simulink model "SAF"  (R2013a)
settings: Solver=ode3  StartTime=0.0  StopTime=0.5  RelTol=1e-3
InitFcn:
  | Ts=5e-6;
libraries: powerlib x25, dsparch4 x1
settings Model: Creator=smartworld  LastModifiedBy=Shubashini
settings DataIOCC: SignalLoggingSaveFormat=ModelDataLogs  InspectSignalLogs=on
settings OptimizationCC: ExpressionDepthLimit=2147483647
settings DebuggingCC: FcnCallInpInsideContextMsg=UseLocalSettings  StrictBusMsg=Warning
settings GRTTargetCC: CombineOutputUpdateFcns=off  GRTInterface=on

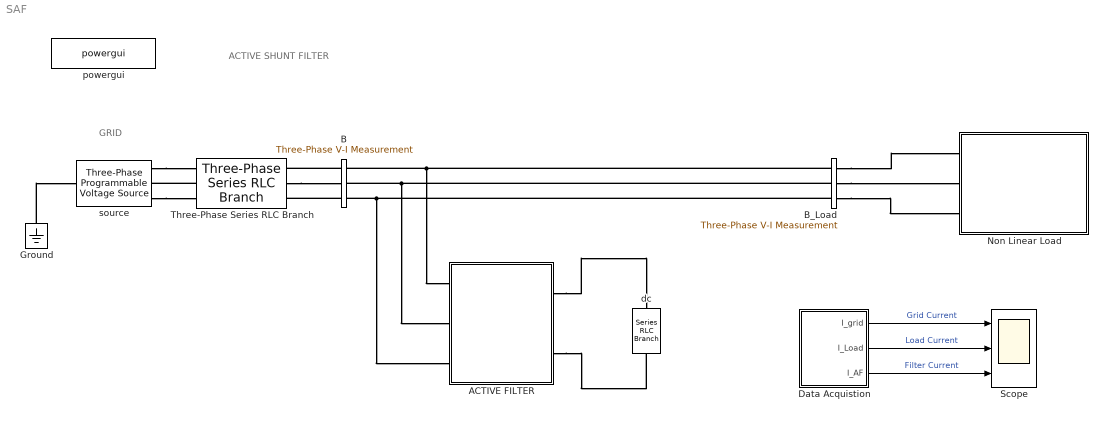
== system SAF ==
  note: ACTIVE SHUNT FILTER
  note: GRID
  ACTIVE FILTER : Subsystem
      mask Display: fprintf('ACTIVE\nFILTER')
  B : powerlib/Measurements/Three-Phase V-I Measurement  VoltageMeasurement=phase-to-ground  SetLabelV=on  LabelV=Vabc  Vpu=off  VpuLL=off  CurrentMeasurement=yes  SetLabelI=on  LabelI=Iabc  Ipu=off  Pbase=100e6  Vbase=500e3  OutputType=Complex  PhasorSimulation=off  PSBequivalent=0
  B_Load : powerlib/Measurements/Three-Phase V-I Measurement  VoltageMeasurement=phase-to-ground  SetLabelV=on  LabelV=Vabc_NL  Vpu=off  VpuLL=off  CurrentMeasurement=yes  SetLabelI=on  LabelI=Iabc_NL  Ipu=off  Pbase=100e6  Vbase=500e3  OutputType=Complex  PhasorSimulation=off  PSBequivalent=0
  Data Acquistion : Subsystem
  Ground : powerlib/Elements/Ground  LConnTagsString=a
  Non Linear Load : Subsystem
      mask Display: fprintf('Non Linear\nLoad')
  Scope : Scope  NumInputPorts=3
      settings: TimeRange=0.5  YMin=-4~-4~-2  YMax=4~4~2  SaveName=Current_pi
  Three-Phase Series RLC Branch : powerlib/Elements/Three-Phase Series RLC Branch  LConnTagsString=A|B|C  RConnTagsString=A|B|C  BranchType=RL  Resistance=0.1  Inductance=0.15e-3  Capacitance=1e-6  Measurements=None
  dc : powerlib/Elements/Series RLC Branch  LConnTagsString=__new0  RConnTagsString=__new0  BranchType=C  Resistance=1  Inductance=1e-3  SetiL0=off  InitialCurrent=0  Capacitance=35e-6  Setx0=off  InitialVoltage=0  Measurements=None
  powergui : powerlib/powergui  Priority=1  SimulationMode=Discrete  SolverType=Tustin  SampleTime=Ts  frequency=60  SPID=off  DisableSnubberDevices=off  DisableRonSwitches=off  DisableVfSwitches=off  SwTol=0  Interpol=off  DisplayEquations=off  frequencyindice=0  Pbase=100e6  ErrMax=1e-4  Iterations=50  UnitsV=kV  UnitsW=MW  FunctionMessages=off  echomessages=off  HookPort=off  EnableUseOfTLC=off  x0status=blocks  RestoreLinks=warning  ResistiveCurrentMeasurement=off  Frange=[0:2:500]  Ylog=on  Xlog=off  ShowGrid=on  save=off  variable=ZData  structure=Current_pi  ZoomFFT=off  StartTime=0.42  cycles=1  DisplayStyle=1  fundamental=50  FreqAxis=off  MaxFrequency=2000  frequencyindicesteady=1  RmsSteady=1  display=off  Ts=0  methode=off
  "source " : powerlib/Electrical Sources/Three-Phase Programmable Voltage Source  PositiveSequence="[100*sqrt(3/2)  0 50]"  VariationEntity=None  VariationType=Step  VariationTypeAlt=Step  VariationStep=0.5  VariationRate=10  VariationMagnitude=0.3  VariationFrequency=2  VariationTiming=[1 2]  VariationPhaseA=off  Amplitudes=[1 0.8 1.2 1.0]  TimeValues=[0 0.1 0.15 0.2]  HarmonicGeneration=off  HarmonicA=[3 0.2 -25 0]  HarmonicB=[2 0.15 35 2]  Timing="[0.05  3]"  BusType=swing  Pref=0  Qref=0  Qmin=-inf  Qmax=inf
  wires:
  Data Acquistion/1(I_grid) -> Scope/1  "Grid Current"
  Data Acquistion/2(I_Load) -> Scope/2  "Load Current"
  Data Acquistion/3(I_AF) -> Scope/3  "Filter Current"
  connections:
  Ground/LConn1 -- "source "/LConn1
  "source "/RConn1 -- Three-Phase Series RLC Branch/LConn1
  Three-Phase Series RLC Branch/LConn2 -- "source "/RConn2
  "source "/RConn3 -- Three-Phase Series RLC Branch/LConn3
  B/LConn1 -- Three-Phase Series RLC Branch/RConn1
  Three-Phase Series RLC Branch/RConn2 -- B/LConn2
  B/LConn3 -- Three-Phase Series RLC Branch/RConn3
  B_Load/LConn1 -- B/RConn1 -- ACTIVE FILTER/RConn1
  B_Load/LConn2 -- B/RConn2 -- ACTIVE FILTER/RConn2
  B_Load/LConn3 -- B/RConn3 -- ACTIVE FILTER/RConn3
  B_Load/RConn3 -- Non Linear Load/LConn3
  B_Load/RConn2 -- Non Linear Load/LConn2
  B_Load/RConn1 -- Non Linear Load/LConn1
  ACTIVE FILTER/LConn1 -- dc/LConn1
  ACTIVE FILTER/LConn2 -- dc/RConn1

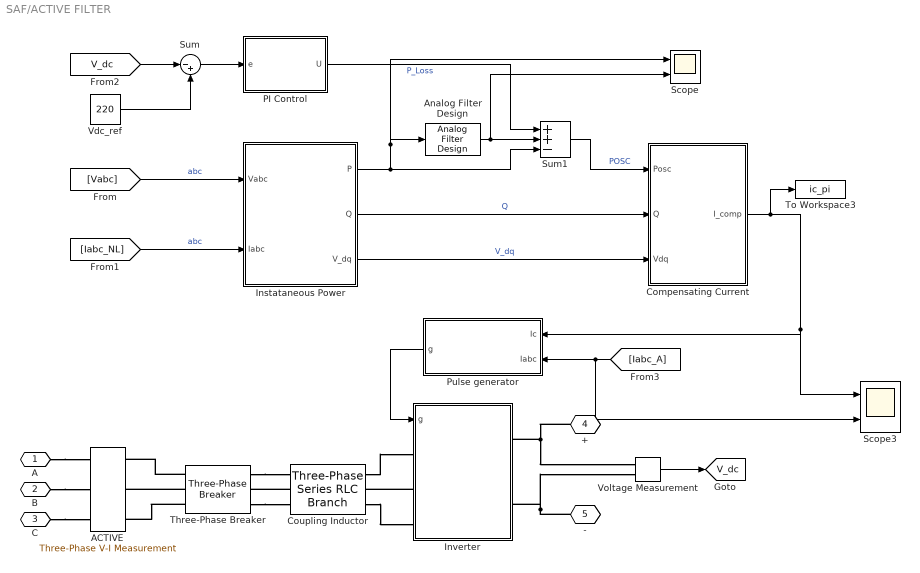
== system SAF/ACTIVE FILTER ==
  ACTIVE : powerlib/Measurements/Three-Phase V-I Measurement  VoltageMeasurement=no  SetLabelV=off  LabelV=Vabc  Vpu=off  VpuLL=off  CurrentMeasurement=yes  SetLabelI=on  LabelI=Iabc_A  Ipu=off  Pbase=100e6  Vbase=500e3  OutputType=Complex  PhasorSimulation=off  PSBequivalent=0
  Analog Filter Design : dsparch4/Analog Filter Design  method=Butterworth  filttype=Lowpass  N=5  Wlo=2*pi*50  Whi=80  Rp=2  Rs=40
  Compensating Current : Subsystem
  Coupling Inductor : powerlib/Elements/Three-Phase Series RLC Branch  LConnTagsString=A|B|C  RConnTagsString=A|B|C  BranchType=L  Resistance=0.001  Inductance=15e-3  Capacitance=1e-6  Measurements=None
  Instataneous Power : Subsystem
  Inverter : Subsystem
  PI Control : Subsystem
      mask Display: fprintf('PI\nControl')
  Pulse generator : Subsystem
      mask Display: fprintf('Pulse\nGenerator')
  Scope : Scope  NumInputPorts=2
      settings: YMin=225~283.75  YMax=325~287.75  SaveName=ScopeData7
  Scope3 : Scope  NumInputPorts=2
      settings: TimeRange=0.5  YMin=-2~-5  YMax=2~6.5  SaveName=ScopeData8
  Sum : Sum  Inputs=|-+
  Sum1 : Sum  Inputs=++-
  Three-Phase Breaker : powerlib/Elements/Three-Phase Breaker  InitialState=closed  SwitchA=on  SwitchB=on  SwitchC=on  SwitchTimes="[0  2/50]"  External=off  BreakerResistance=0.001  SnubberResistance=1e6  SnubberCapacitance=inf  Measurements=None
  To Workspace3 : ToWorkspace  VariableName=ic_pi  SampleTime=Ts
  Vdc_ref : Constant  Value=220
  Voltage Measurement : powerlib/Measurements/Voltage Measurement  PhasorSimulation=off  OutputType=Complex  PSBequivalent=0
  A : PMIOPort  Port=1  Side=Right
  B : PMIOPort  Port=2  Side=Right
  C : PMIOPort  Port=3  Side=Right
  + : PMIOPort  Tag=PMCPort  Port=4  Side=Left
  - : PMIOPort  Tag=PMCPort  Port=5  Side=Left
  tag scope: V_dc=global
  wires:
  Voltage Measurement/1 -> [V_dc]
  Vdc_ref/1 -> Sum/2
  Sum/1 -> PI Control/1(e)
  [Vabc] -> Instataneous Power/1(Vabc)  "abc"
  [Iabc_NL] -> Instataneous Power/2(Iabc)  "abc"
  Instataneous Power/1(P) -> Sum1/3, Analog Filter Design/1, Scope/1
  [V_dc] -> Sum/1
  Analog Filter Design/1 -> Sum1/2, Scope/2
  PI Control/1(U) -> Sum1/1  "P_Loss"
  Sum1/1 -> Compensating Current/1(Posc)  "POSC"
  Instataneous Power/2(Q) -> Compensating Current/2(Q)  "Q"
  Instataneous Power/3(V_dq) -> Compensating Current/3(Vdq)  "V_dq"
  Compensating Current/1(I_comp) -> To Workspace3/1, Pulse generator/1(Ic), Scope3/1
  [Iabc_A] -> Pulse generator/2(Iabc), Scope3/2
  Pulse generator/1(g) -> Inverter/1(g)
  connections:
  Inverter/LConn2 -- Coupling Inductor/RConn2
  A/RConn1 -- ACTIVE/RConn1
  B/RConn1 -- ACTIVE/RConn2
  C/RConn1 -- ACTIVE/RConn3
  Three-Phase Breaker/RConn1 -- Coupling Inductor/LConn1
  Coupling Inductor/LConn2 -- Three-Phase Breaker/RConn2
  Three-Phase Breaker/RConn3 -- Coupling Inductor/LConn3
  Three-Phase Breaker/LConn3 -- ACTIVE/LConn3
  Three-Phase Breaker/LConn2 -- ACTIVE/LConn2
  Three-Phase Breaker/LConn1 -- ACTIVE/LConn1
  Coupling Inductor/RConn1 -- Inverter/LConn1
  Coupling Inductor/RConn3 -- Inverter/LConn3
  +/RConn1 -- Inverter/RConn1 -- Voltage Measurement/LConn1
  -/RConn1 -- Inverter/RConn2 -- Voltage Measurement/LConn2

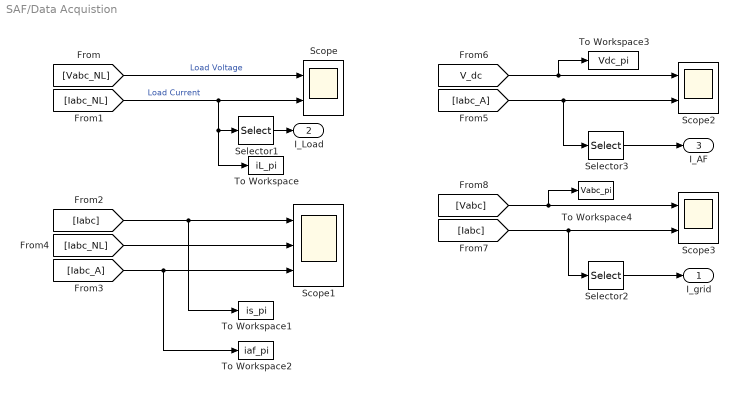
== system SAF/Data Acquistion ==
  Scope : Scope  NumInputPorts=2
      settings: TimeRange=0.5  YMin=-100~-20  YMax=100~20
  Scope1 : Scope  NumInputPorts=3
      settings: TimeRange=0.5  YMin=-10~-3~-6  YMax=10~3~8  SaveName=ScopeData2
  Scope2 : Scope  NumInputPorts=2
      settings: TimeRange=0.5  YMin=-50~-6  YMax=350~8
  Scope3 : Scope  NumInputPorts=2
      settings: TimeRange=1  YMin=-150~-10  YMax=150~8  SaveName=ScopeData6
  Selector1 : Selector  InputPortWidth=3  IndexOptions=Index vector (dialog)  Indices=1  OutputSizes=1
  Selector2 : Selector  InputPortWidth=3  IndexOptions=Index vector (dialog)  Indices=1  OutputSizes=1
  Selector3 : Selector  InputPortWidth=3  IndexOptions=Index vector (dialog)  Indices=1  OutputSizes=1
  To Workspace : ToWorkspace  VariableName=iL_pi  SampleTime=Ts
  To Workspace1 : ToWorkspace  VariableName=is_pi  SampleTime=Ts
  To Workspace2 : ToWorkspace  VariableName=iaf_pi  SampleTime=Ts
  To Workspace3 : ToWorkspace  VariableName=Vdc_pi  SampleTime=Ts
  To Workspace4 : ToWorkspace  VariableName=Vabc_pi  SampleTime=Ts
  I_grid : Outport
  I_Load : Outport  Port=2
  I_AF : Outport  Port=3
  wires:
  [Vabc_NL] -> Scope/1  "Load Voltage"
  [Iabc_NL] -> Scope/2, Selector1/1, To Workspace/1  "Load Current"
  [Iabc] -> Scope1/1, To Workspace1/1
  [Iabc_NL] -> Scope1/2
  [Iabc_A] -> Scope1/3, To Workspace2/1
  Selector1/1 -> I_Load/1
  [Iabc_A] -> Scope2/2, Selector3/1
  [V_dc] -> Scope2/1, To Workspace3/1
  Selector3/1 -> I_AF/1
  [Iabc] -> Scope3/2, Selector2/1
  [Vabc] -> Scope3/1, To Workspace4/1
  Selector2/1 -> I_grid/1

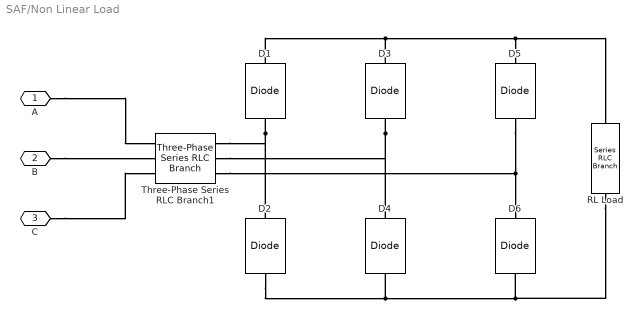
== system SAF/Non Linear Load ==
  D{1..6} (6 alike) : powerlib/Power Electronics/Diode  Ron=0.001  Lon=0  Vf=0.8  IC=0  UseSnubber=off  Rs=500  Cs=250e-9  Measurements=off
  RL Load : powerlib/Elements/Series RLC Branch  LConnTagsString=__new0  RConnTagsString=__new0  BranchType=RL  Resistance=60  Inductance=20e-3  SetiL0=off  InitialCurrent=0  Capacitance=1e-6  Setx0=off  InitialVoltage=0  Measurements=None
  Three-Phase Series RLC Branch1 : powerlib/Elements/Three-Phase Series RLC Branch  LConnTagsString=A|B|C  RConnTagsString=A|B|C  BranchType=RL  Resistance=0.4  Inductance=3.55e-3  Capacitance=1e-6  Measurements=None
  A : PMIOPort  Port=1  Side=Left
  B : PMIOPort  Port=2  Side=Left
  C : PMIOPort  Port=3  Side=Left
  connections:
  D1/LConn1 -- D2/RConn1 -- Three-Phase Series RLC Branch1/RConn1
  D1/RConn1 -- D3/RConn1 -- D5/RConn1 -- RL Load/LConn1
  D2/LConn1 -- D4/LConn1 -- D6/LConn1 -- RL Load/RConn1
  D3/LConn1 -- D4/RConn1 -- Three-Phase Series RLC Branch1/RConn2
  D5/LConn1 -- D6/RConn1 -- Three-Phase Series RLC Branch1/RConn3
  A/RConn1 -- Three-Phase Series RLC Branch1/LConn1
  B/RConn1 -- Three-Phase Series RLC Branch1/LConn2
  C/RConn1 -- Three-Phase Series RLC Branch1/LConn3

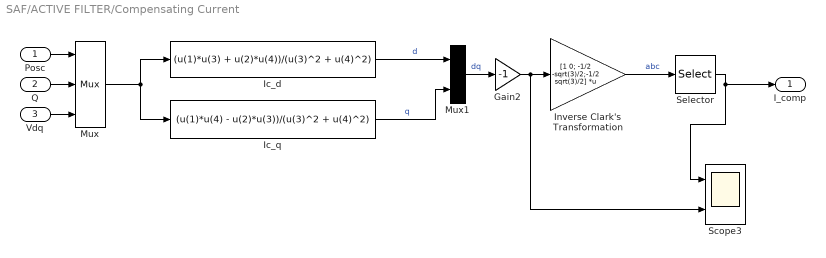
== system SAF/ACTIVE FILTER/Compensating Current ==
  Posc : Inport
  Q : Inport  Port=2
  Vdq : Inport  Port=3
  Gain2 : Gain  Gain=-1
  "Ic_d " : Fcn  Expr=(u(1)*u(3) + u(2)*u(4))/(u(3)^2 + u(4)^2)
  Ic_q : Fcn  Expr=(u(1)*u(4) - u(2)*u(3))/(u(3)^2 + u(4)^2)
  Inverse Clark's Transformation : Gain  Gain=[1 0; -1/2 -sqrt(3)/2;-1/2 sqrt(3)/2]  Multiplication=Matrix(K*u)
  Mux : Mux  Inputs=3
      settings: DisplayOption=signals
  Mux1 : Mux  Inputs=2
      settings: DisplayOption=signals
  Scope3 : Scope  NumInputPorts=2
      settings: TimeRange=0.5  YMin=-1~-1  YMax=0.6~1  SaveName=ScopeData3
  Selector : Selector  InputPortWidth=3  IndexOptions=Index vector (dialog)  Indices=[1 3 2]  OutputSizes=1
  I_comp : Outport
  wires:
  Posc/1 -> Mux/1
  Q/1 -> Mux/2
  Vdq/1 -> Mux/3
  Mux1/1 -> Gain2/1  "dq"
  Inverse Clark's Transformation/1 -> Selector/1  "abc"
  Mux/1 -> Ic_q/1, "Ic_d "/1
  "Ic_d "/1 -> Mux1/1  "d"
  Ic_q/1 -> Mux1/2  "q"
  Selector/1 -> I_comp/1, Scope3/1
  Gain2/1 -> Inverse Clark's Transformation/1, Scope3/2

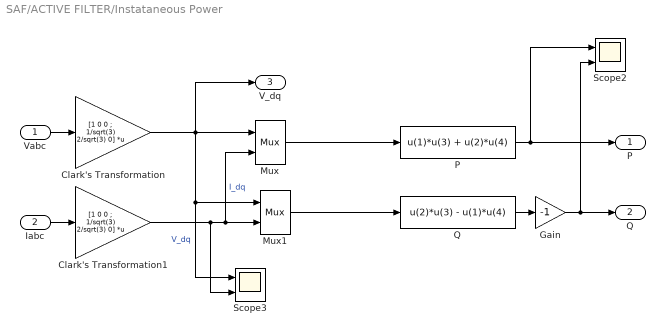
== system SAF/ACTIVE FILTER/Instataneous Power ==
  Vabc : Inport
  Iabc : Inport  Port=2
  " Q" : Fcn  Expr=u(2)*u(3) - u(1)*u(4)
  Clark's Transformation : Gain  Gain=[1 0 0 ; 1/sqrt(3) 2/sqrt(3) 0]  Multiplication=Matrix(K*u)
  Clark's Transformation1 : Gain  Gain=[1 0 0 ; 1/sqrt(3) 2/sqrt(3) 0]  Multiplication=Matrix(K*u)
  Gain : Gain  Gain=-1
  Mux : Mux  Inputs=2
      settings: DisplayOption=signals
  Mux1 : Mux  Inputs=2
      settings: DisplayOption=signals
  "P " : Fcn  Expr=u(1)*u(3) + u(2)*u(4)
  Scope2 : Scope  NumInputPorts=2
      settings: TimeRange=0.5  YMin=5~-20  YMax=35~15  SaveName=ScopeData4
  Scope3 : Scope  NumInputPorts=2
      settings: TimeRange=1  YMin=-100~-3  YMax=100~3  SaveName=ScopeData5
  P : Outport
  Q : Outport  Port=2
  V_dq : Outport  Port=3
  wires:
  Clark's Transformation1/1 -> Mux/2, Mux1/2, Scope3/2  "I_dq"
  Clark's Transformation/1 -> Mux/1, V_dq/1, Mux1/1, Scope3/1  "V_dq"
  Mux/1 -> "P "/1
  Mux1/1 -> " Q"/1
  Vabc/1 -> Clark's Transformation/1
  " Q"/1 -> Gain/1
  Iabc/1 -> Clark's Transformation1/1
  "P "/1 -> P/1, Scope2/1
  Gain/1 -> Q/1, Scope2/2

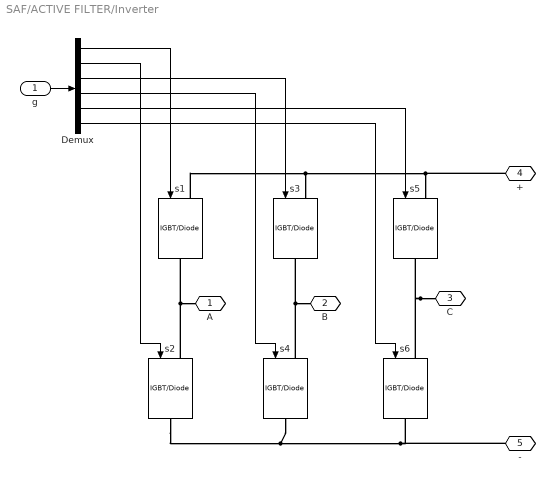
== system SAF/ACTIVE FILTER/Inverter ==
  g : Inport
  Demux : Demux  Outputs=6
  s{1..6} (6 alike) : powerlib/Power Electronics/IGBT//Diode  Ron=1e-3  Rs=1e5  Cs=inf  Measurements=off
  A : PMIOPort  Port=1  Side=Left
  B : PMIOPort  Port=2  Side=Left
  C : PMIOPort  Port=3  Side=Left
  + : PMIOPort  Port=4  Side=Right
  - : PMIOPort  Port=5  Side=Right
  wires:
  g/1 -> Demux/1
  Demux/1 -> s1/1
  Demux/2 -> s2/1
  Demux/3 -> s3/1
  Demux/4 -> s4/1
  Demux/5 -> s5/1
  Demux/6 -> s6/1
  connections:
  s1/LConn1 -- s3/LConn1 -- s5/LConn1 -- +/RConn1
  A/RConn1 -- s2/LConn1 -- s1/RConn1
  s2/RConn1 -- s4/RConn1 -- s6/RConn1 -- -/RConn1
  B/RConn1 -- s4/LConn1 -- s3/RConn1
  C/RConn1 -- s6/LConn1 -- s5/RConn1

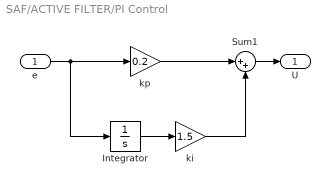
== system SAF/ACTIVE FILTER/PI Control ==
  e : Inport
  Integrator : Integrator
  Sum1 : Sum  Inputs=|++
  ki : Gain  Gain=1.5
  kp : Gain  Gain=0.2
  U : Outport
  wires:
  kp/1 -> Sum1/1
  ki/1 -> Sum1/2
  Integrator/1 -> ki/1
  e/1 -> kp/1, Integrator/1
  Sum1/1 -> U/1

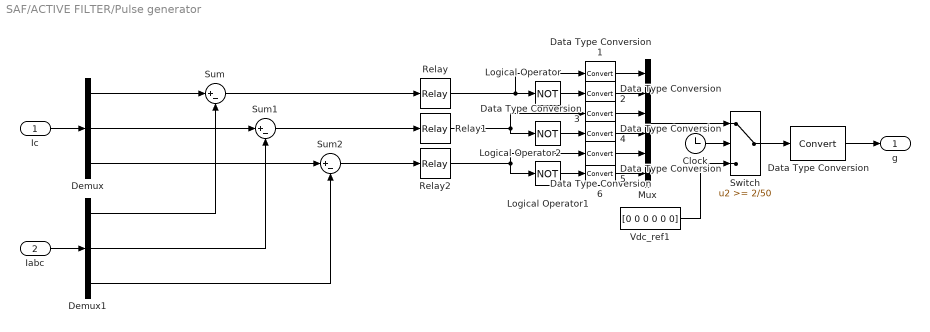
== system SAF/ACTIVE FILTER/Pulse generator ==
  Ic : Inport
  Iabc : Inport  Port=2
  Clock : Clock
  Data Type Conversion{,1..6} (7 alike) : DataTypeConversion
  Demux : Demux  Outputs=3
  Demux1 : Demux  Outputs=3
  Logical Operator : Logic  Operator=NOT  AllPortsSameDT=off  OutDataTypeStr=boolean
  Logical Operator1 : Logic  Operator=NOT  AllPortsSameDT=off  OutDataTypeStr=boolean
  Logical Operator2 : Logic  Operator=NOT  AllPortsSameDT=off  OutDataTypeStr=boolean
  Mux : Mux  Inputs=6
  Relay : Relay  OnSwitchValue=0.02  OffSwitchValue=-0.02
  Relay1 : Relay  OnSwitchValue=0.02  OffSwitchValue=-0.02
  Relay2 : Relay  OnSwitchValue=0.02  OffSwitchValue=-0.02
  Sum : Sum  Inputs=|+-
  Sum1 : Sum  Inputs=|+-
  Sum2 : Sum  Inputs=|+-
  Switch : Switch  Threshold=2/50
  Vdc_ref1 : Constant  Value=[0 0 0 0 0 0]
  g : Outport
  wires:
  Ic/1 -> Demux/1
  Demux/1 -> Sum/1
  Demux/2 -> Sum1/1
  Demux/3 -> Sum2/1
  Iabc/1 -> Demux1/1
  Demux1/1 -> Sum/2
  Demux1/2 -> Sum1/2
  Demux1/3 -> Sum2/2
  Sum/1 -> Relay/1
  Sum1/1 -> Relay1/1
  Sum2/1 -> Relay2/1
  Data Type Conversion/1 -> g/1
  Clock/1 -> Switch/2
  Relay/1 -> Logical Operator/1, Data Type Conversion1/1
  Relay2/1 -> Logical Operator1/1, Data Type Conversion6/1
  Logical Operator1/1 -> Data Type Conversion5/1
  Logical Operator/1 -> Data Type Conversion2/1
  Relay1/1 -> Logical Operator2/1, Data Type Conversion3/1
  Logical Operator2/1 -> Data Type Conversion4/1
  Data Type Conversion1/1 -> Mux/1
  Data Type Conversion2/1 -> Mux/2
  Data Type Conversion3/1 -> Mux/3
  Data Type Conversion4/1 -> Mux/4
  Data Type Conversion5/1 -> Mux/6
  Data Type Conversion6/1 -> Mux/5
  Mux/1 -> Switch/1
  Switch/1 -> Data Type Conversion/1
  Vdc_ref1/1 -> Switch/3
